simulink model "BLDC_120deg_LUT"  (R2024a)
settings: Solver=ode15s  StartTime=0.0  StopTime=1.5  RelTol=1e-3
model workspace (MAT data in the model file):
  t = 3
values from neighbouring files (symbols this model uses):
  D_m = 1e-3    (= 0.001)    [BLDC_Parameters.m]
  J_t = 1e-3    (= 0.001)    [BLDC_Parameters.m]
  L_ss = tau_s * r_s    (= 0.0003657)    [BLDC_Parameters.m]
  lambda_m = torque_const/(3*P/4)    (= 0.00985)    [BLDC_Parameters.m]
  omega = out.omega(end)    [filter.m]
  P = 8    [BLDC_Parameters.m]
  r_s = r_pp/2    (= 0.345)    [BLDC_Parameters.m]
  R_vs = 1e6    (= 1000000)    [BLDC_Parameters.m]
  tau_s = 1.06e-3    (= 0.00106)    [BLDC_Parameters.m]
  V_bus = 12    [BLDC_Parameters.m]
undefined symbols (not defined in the file or in its folder): HallError1, HallError2, HallError3, tau_corr1, WrappedHallError1
libraries: simulink x14, spsMosfetLib x6, spsSeriesRLCBranchLib x4, spsVoltageMeasurementLib x3, spsControlledCurrentSourceLib x3, slpidlib x1, spsPWMGeneratorDCDCLib x1, spsDCVoltageSourceLib x1, sps_lib x1
settings Model: Creator=matthewhasman  LastModifiedBy=matthewhasman

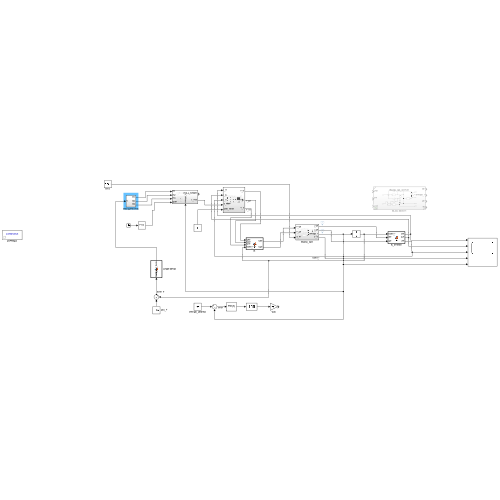
[thumbnail: Simulink's stored preview of the top-level diagram]
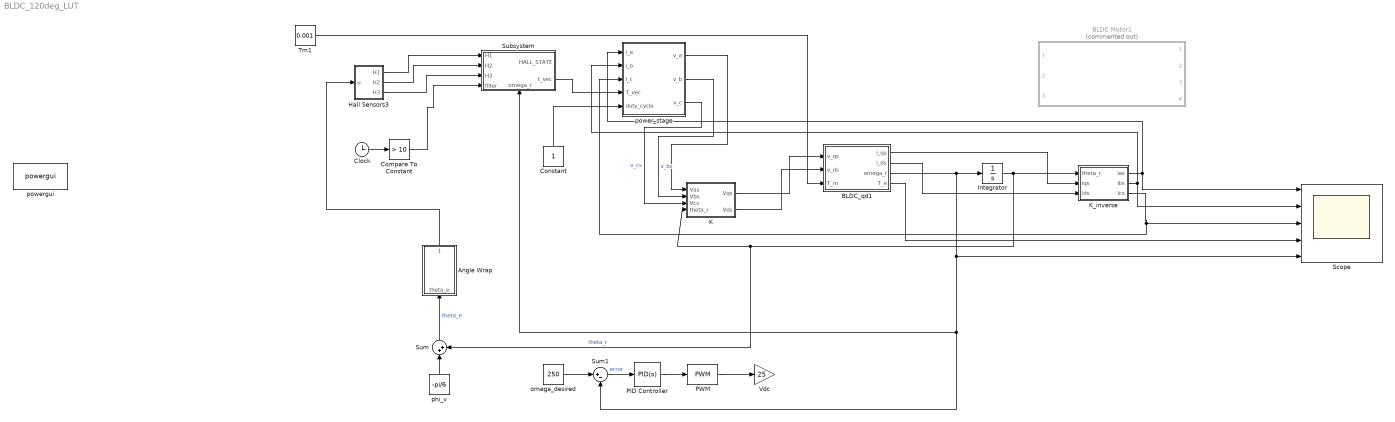
== system BLDC_120deg_LUT ==
  Angle Wrap : MATLAB Function  TreatAsAtomicUnit=on
  BLDC Motor1 : Subsystem  Commented=on  ReferencedSubsystem=BLDC_qd_coords
  BLDC_qd1 : Subsystem
  Clock : Clock
  Compare To Constant : simulink/Logic and Bit Operations/Compare To Constant  relop=>  const=10  OutDataTypeStr=boolean
  Constant : Constant
  Hall Sensors3 : Subsystem
  Integrator : Integrator
  K : MATLAB Function  TreatAsAtomicUnit=on
  K_inverse : MATLAB Function  TreatAsAtomicUnit=on
  PID Controller : slpidlib/PID Controller  Controller=PID  Form=Parallel  TimeDomain=Continuous-time  UseExternalTs=off  SampleTime=-1  IntegratorMethod=Forward Euler  FilterMethod=Forward Euler  ControllerParametersSource=internal  P=8  I=5  UseKiTs=off  D=1  UseExternalDerivativeSource=off  N=100  UseFilter=on  TunerSelectOption=Transfer Function Based (PID Tuner App)  InitialConditionSource=internal  InitialConditionForIntegrator=0  InitialConditionForFilter=0  DifferentiatorICPrevScaledInput=0  ExternalReset=none  TrackingMode=off  Kt=1  LimitOutput=off  SatLimitsSource=internal  UpperSaturationLimit=inf  LowerSaturationLimit=-inf  LinearizeAsGain=on  AntiWindupMode=none  Kb=1  LimitIntegrator=off  UpperIntegratorSaturationLimit=inf  LowerIntegratorSaturationLimit=-inf  POutMin=[]  POutMax=[]  IOutMin=[]  IOutMax=[]  DOutMin=[]  DOutMax=[]  NOutMin=[]  NOutMax=[]  SumOutMin=[]  SumOutMax=[]  SaturationOutMin=[]  SaturationOutMax=[]  PParamMin=[]  PParamMax=[]  IParamMin=[]  IParamMax=[]  DParamMin=[]  DParamMax=[]  NParamMin=[]  NParamMax=[]  KbParamMin=[]  KbParamMax=[]  KtParamMin=[]  KtParamMax=[]  KbOutMin=[]  KbOutMax=[]  KtOutMin=[]  KtOutMax=[]  IntegratorOutMin=[]  IntegratorOutMax=[]  FilterOutMin=[]  FilterOutMax=[]  SumI1OutMin=[]  SumI1OutMax=[]  SumI2OutMin=[]  SumI2OutMax=[]  SumI3OutMin=[]  SumI3OutMax=[]  SumI4OutMin=[]  SumI4OutMax=[]  SumDOutMin=[]  SumDOutMax=[]  DifferentiatorOutMin=[]  DifferentiatorOutMax=[]  FilterDiffOutCoefMin=[]  FilterDiffOutCoefMax=[]  ReciprocalOutMin=[]  ReciprocalOutMax=[]  SumDenOutMin=[]  SumDenOutMax=[]  SumNumOutMin=[]  SumNumOutMax=[]  DivideOutMin=[]  DivideOutMax=[]  UdiffTsProdOutMin=[]  UdiffTsProdOutMax=[]  NTsProdOutMin=[]  NTsProdOutMax=[]  UintegralTsProdOutMin=[]  UintegralTsProdOutMax=[]  UngainTsProdOutMin=[]  UngainTsProdOutMax=[]  ClampingZeroOutDataTypeStr=Inherit: Inherit via back propagation  ClampingZeroOutMin=[]  ClampingZeroOutMax=[]  FilterDenConstantOutDataTypeStr=Inherit: Inherit via back propagation  FilterDenConstantOutMin=[]  FilterDenConstantOutMax=[]  PCopyOutDataTypeStr=Inherit: Inherit via back propagation  PCopyOutMin=[]  PCopyOutMax=[]  NCopyOutDataTypeStr=Inherit: Inherit via back propagation  NCopyOutMin=[]  NCopyOutMax=[]  IntegratorContinuousStateAttributes=''  IntegratorStateMustResolveToSignalObject=off  IntegratorRTWStateStorageClass=Auto  FilterContinuousStateAttributes=''  FilterStateMustResolveToSignalObject=off  FilterRTWStateStorageClass=Auto  ParallelPVariant=InternalParameters  IdealPVariant=Disabled  IVariant=InternalParameters  DVariant=InternalParameters  IntegratorVariant=Continuous  SatVariant=Disabled  AWVariant=Passthrough  PCopyVariant=Disabled  TRVariant=Disabled  FdbkBlocksVariant=Forward  IdealPFdbkVariant=Disabled  SatFdbkVariant=Disabled  DerivativeFilterVariant=ContFilter  NVariant=InternalParameters  NCopyVariant=Disabled  FilterICVariant=InternalICsFilter  IntegratorICVariant=InternalICs  ExternalResetVariant=Disabled  TRSumVariant=Passthrough  SumFdbkVariant=Disabled  SumVariant=Sum_PID  TsampFilterVariant=InternalTs  TsampNgainVariant=Passthrough  TsampIntegralVariant=Disabled_SignalSpec  ExternalSaturationOutDataTypeStr=Inherit: Same as second input  DerivativeSourceVariant=ErrorSignal
  PWM : simulink/Discontinuities/PWM  DisableCoverage=on  Period=0.0001  InitialDelay=0  DisallowZeroDutyCycle=off  RunAtFixedTimeIntervals=off  SampleTime=0.1
  Scope : Scope  NumInputPorts=5
  Subsystem : Subsystem
      settings: PortSchema="{\"entries\":[{\"content\":{\"sides\":[{\"content\":{\"connectorIds\":[\"In1\",\"In2\",\"In3\",\"In4\"]},\"type\":\"ConnectorPlacement.EquallySpacedRectSide\",\"uuid\":\"971d0d47-82fe-4afe-af38-e6db618daf70\"},{\"content\":{\"connectorIds\":[\"Out1\",\"Out2\"],\"side\":\"RIGHT\"},\"type\":\"ConnectorPlacement.EquallySpacedRectSide\",\"uuid\":\"04121426-e5e1-4fdf-a823-1b0728fc829c\"},{\"content\":{\"side\":\"TOP\"},\"type\":\"ConnectorPlacement.EquallySpacedRectSide\",\"uuid\":\"8184400a-788f-412d-9776-29e4a0174c8c\"},{\"content\":{\"connectorIds\":[\"In5\"],\"side\":\"BOTTOM\"},\"type\":\"ConnectorPlacement.EquallySpacedRectSide\",\"uuid\":\"7ee8c5a1-7866-4d62-ba50-cd64eb02da7d\"}]},\"type\":\"ConnectorPlacement.EquallySpacedConnector\",\"uuid\":\"0b8e8def-6998-42e4-af89-aa5c552bf5ba\"}],\"packageUris\":[\"http://schema.mathworks.com/mf0/Connector/R2020b\"],\"version\":\"1.0\"}"
  Sum : Sum  Inputs=|++
  Sum1 : Sum  Inputs=|+-
  Tm1 : Constant  Value=0.001
  Vdc : Gain  Gain=25
  omega_desired : Constant  Value=250
  phi_v : Constant  Value=-pi/6
  power_stage : Subsystem
  powergui : sps_lib/powergui  Priority=1  SimulationMode=Continuous  SampleTime=50e-6  frequency=60  Iterations=50  frequencyindice=0  Pbase=100e6  ErrMax=1e-4  UnitsV=kV  UnitsW=MW  buscounter=0  FunctionMessages=off  echomessages=off  EnableUseOfTLC=off  CurrentSourceSwitches=off  DisableSnubberDevices=off  DisableRonSwitches=off  DisableVfSwitches=off  DisplayEquations=off  AutomaticDiscreteSolvers=off  SolverType=Tustin/Backward Euler (TBE)  Interpol=off  ExternalGateDelay=off  methode=off  Ts=100  x0status=blocks  SPID=on  SwTol=0  HookPort=off  NonlinearTolerance=1e-4  nMaxIteration=100  ContinueOnMaxIteration=off  RestoreLinks=warning  ResistiveCurrentMeasurement=off  Frange=[0:2:500]  Ylog=off  Xlog=on  ShowGrid=off  save=off  variable=ZData  structure=0  ZoomFFT=off  StartTime=0.0  cycles=1  DisplayStyle=1  fundamental=60  FreqAxis=off  MaxFrequency=1000  frequencyindicesteady=1  RmsSteady=1  display=off
  wires:
  Integrator/1 -> K_inverse/1(theta_r), K/4(theta_r), Sum/2  "theta_r"
  BLDC_qd1/1(i_qs) -> K_inverse/2(iqs)
  BLDC_qd1/2(i_ds) -> K_inverse/3(ids)
  K/1(Vqs) -> BLDC_qd1/1(v_qs)
  Tm1/1 -> BLDC_qd1/3(T_m)
  phi_v/1 -> Sum/1
  omega_desired/1 -> Sum1/1
  Sum1/1 -> PID Controller/1  "error"
  PID Controller/1 -> PWM/1
  PWM/1 -> Vdc/1
  K/2(Vds) -> BLDC_qd1/2(v_ds)
  Sum/1 -> Angle Wrap/1(theta_e)  "theta_e"
  BLDC_qd1/3(omega_r) -> Subsystem/5(omega_r), Sum1/2, Scope/5, Integrator/1
  BLDC_qd1/4(T_e) -> Scope/4
  K_inverse/1(ias) -> power_stage/1(i_a), Scope/1
  K_inverse/2(ibs) -> power_stage/2(i_b), Scope/2
  K_inverse/3(ics) -> power_stage/3(i_c), Scope/3
  Constant/1 -> power_stage/5(duty_cycle)
  power_stage/1(v_a) -> K/1(Vas)
  power_stage/2(v_b) -> K/2(Vbs)  "v_bs"
  power_stage/3(v_c) -> K/3(Vcs)  "v_cs"
  Angle Wrap/1(wrapped_theta) -> Hall Sensors3/1(u)
  Clock/1 -> Compare To Constant/1
  Hall Sensors3/1(H1) -> Subsystem/1(H1)
  Hall Sensors3/2(H2) -> Subsystem/2(H2)
  Hall Sensors3/3(H3) -> Subsystem/3(H3)
  Compare To Constant/1 -> Subsystem/4(filter)
  Subsystem/2(t_vec) -> power_stage/4(T_vec)

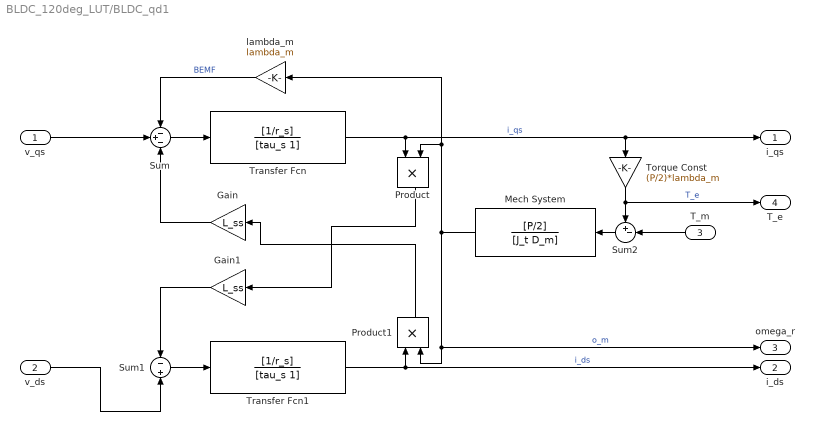
== system BLDC_120deg_LUT/BLDC_qd1 ==
  v_qs : Inport
  v_ds : Inport  Port=2
  T_m : Inport  Port=3
  Gain : Gain  Gain=L_ss
  Gain1 : Gain  Gain=L_ss
  Mech System : TransferFcn  Numerator=[P/2]  Denominator=[J_t D_m]
  Product : Product
  Product1 : Product
  Sum : Sum  Inputs=-+-
  Sum1 : Sum  Inputs=-+
  Sum2 : Sum  Inputs=+-|
  Torque Const : Gain  Gain=(P/2)*lambda_m
  Transfer Fcn : TransferFcn  Numerator=[1/r_s]  Denominator=[tau_s 1]
  Transfer Fcn1 : TransferFcn  Numerator=[1/r_s]  Denominator=[tau_s 1]
  lambda_m : Gain  Gain=lambda_m
  i_qs : Outport
  i_ds : Outport  Port=2
  omega_r : Outport  Port=3
  T_e : Outport  Port=4
  wires:
  T_m/1 -> Sum2/2
  Sum1/1 -> Transfer Fcn1/1
  Gain1/1 -> Sum1/1
  Product1/1 -> Gain/1
  Transfer Fcn1/1 -> i_ds/1, Product1/1  "i_ds"
  Mech System/1 -> lambda_m/1, Product/2, omega_r/1, Product1/2  "o_m"
  Torque Const/1 -> T_e/1, Sum2/1  "T_e"
  v_ds/1 -> Sum1/2
  Transfer Fcn/1 -> i_qs/1, Torque Const/1, Product/1  "i_qs"
  Product/1 -> Gain1/1
  Gain/1 -> Sum/3
  v_qs/1 -> Sum/2
  Sum/1 -> Transfer Fcn/1
  Sum2/1 -> Mech System/1
  lambda_m/1 -> Sum/1  "BEMF"

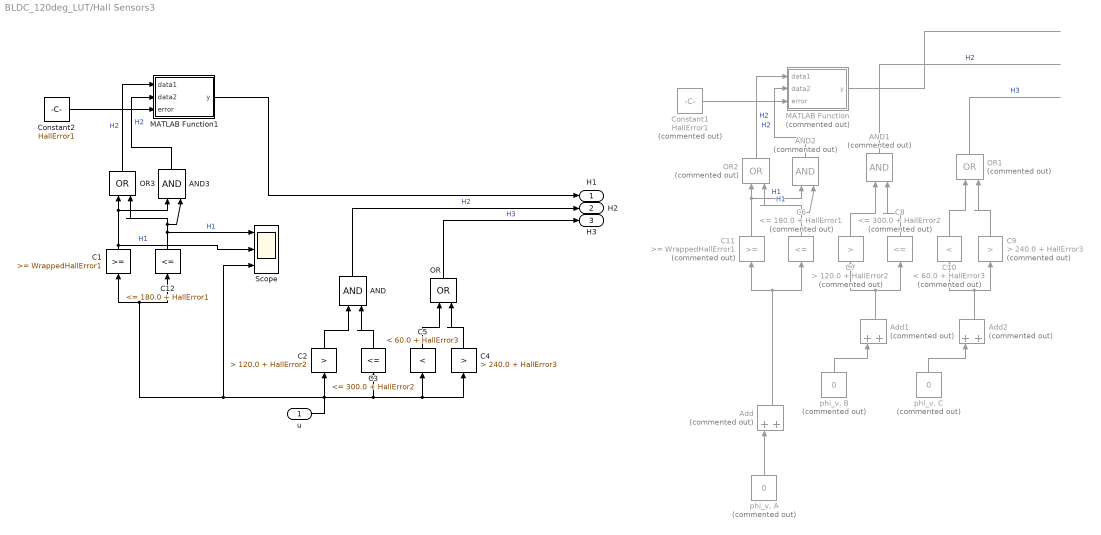
== system BLDC_120deg_LUT/Hall Sensors3 ==
  u : Inport
  AND : Logic  IconShape=distinctive  AllPortsSameDT=off  OutDataTypeStr=boolean
  AND1 : Logic  Commented=on  IconShape=distinctive  AllPortsSameDT=off  OutDataTypeStr=boolean
  AND2 : Logic  Commented=on  IconShape=distinctive  AllPortsSameDT=off  OutDataTypeStr=boolean
  AND3 : Logic  IconShape=distinctive  AllPortsSameDT=off  OutDataTypeStr=boolean
  Add : Sum  Commented=on
  Add1 : Sum  Commented=on
  Add2 : Sum  Commented=on
  C1 : simulink/Logic and Bit Operations/Compare To Constant  relop=>=  const=WrappedHallError1  OutDataTypeStr=boolean
  C10 : simulink/Logic and Bit Operations/Compare To Constant  Commented=on  relop=<  const=60.0 + HallError3  OutDataTypeStr=boolean
  C11 : simulink/Logic and Bit Operations/Compare To Constant  Commented=on  relop=>=  const=WrappedHallError1  OutDataTypeStr=boolean
  C12 : simulink/Logic and Bit Operations/Compare To Constant  relop=<=  const=180.0 + HallError1  OutDataTypeStr=boolean
  C2 : simulink/Logic and Bit Operations/Compare To Constant  relop=>  const=120.0 + HallError2  OutDataTypeStr=boolean
  C3 : simulink/Logic and Bit Operations/Compare To Constant  relop=<=  const=300.0 + HallError2  OutDataTypeStr=boolean
  C4 : simulink/Logic and Bit Operations/Compare To Constant  relop=>  const=240.0 + HallError3  OutDataTypeStr=boolean
  C5 : simulink/Logic and Bit Operations/Compare To Constant  relop=<  const=60.0 + HallError3  OutDataTypeStr=boolean
  C6 : simulink/Logic and Bit Operations/Compare To Constant  Commented=on  relop=<=  const=180.0 + HallError1  OutDataTypeStr=boolean
  C7 : simulink/Logic and Bit Operations/Compare To Constant  Commented=on  relop=>  const=120.0 + HallError2  OutDataTypeStr=boolean
  C8 : simulink/Logic and Bit Operations/Compare To Constant  Commented=on  relop=<=  const=300.0 + HallError2  OutDataTypeStr=boolean
  C9 : simulink/Logic and Bit Operations/Compare To Constant  Commented=on  relop=>  const=240.0 + HallError3  OutDataTypeStr=boolean
  Constant1 : Constant  Commented=on  Value=HallError1
  Constant2 : Constant  Value=HallError1
  MATLAB Function : MATLAB Function  Commented=on  TreatAsAtomicUnit=on
  MATLAB Function1 : MATLAB Function  TreatAsAtomicUnit=on
  OR : Logic  Operator=OR  IconShape=distinctive  AllPortsSameDT=off  OutDataTypeStr=boolean
  OR1 : Logic  Commented=on  Operator=OR  IconShape=distinctive  AllPortsSameDT=off  OutDataTypeStr=boolean
  OR2 : Logic  Commented=on  Operator=OR  IconShape=distinctive  AllPortsSameDT=off  OutDataTypeStr=boolean
  OR3 : Logic  Operator=OR  IconShape=distinctive  AllPortsSameDT=off  OutDataTypeStr=boolean
  Scope : Scope  NumInputPorts=3
  "phi_v, A" : Constant  Commented=on  Value=0
  "phi_v, B" : Constant  Commented=on  Value=0
  "phi_v, C" : Constant  Commented=on  Value=0
  H1 : Outport
  H2 : Outport  Port=2
  H3 : Outport  Port=3
  wires:
  C5/1 -> OR/1
  AND/1 -> H2/1  "H2"
  C4/1 -> OR/2
  C3/1 -> AND/2
  C2/1 -> AND/1
  OR/1 -> H3/1  "H3"
  Add1/1 -> C8/1, C7/1
  "phi_v, C"/1 -> Add2/1
  "phi_v, B"/1 -> Add1/1
  C10/1 -> OR1/1
  ? -> Add2/2, Add1/2, Add/2
  OR2/1 -> MATLAB Function/1(data1)  "H2"
  "phi_v, A"/1 -> Add/1
  C9/1 -> OR1/2
  Add/1 -> C6/1, C11/1
  C7/1 -> AND1/1
  Add2/1 -> C10/1, C9/1
  Constant1/1 -> MATLAB Function/3(error)
  OR1/1 -> ?  "H3"
  AND1/1 -> ?  "H2"
  C6/1 -> AND2/2, OR2/2  "H1"
  AND2/1 -> MATLAB Function/2(data2)  "H2"
  MATLAB Function/1(y) -> ?
  C11/1 -> AND2/1, OR2/1  "H1"
  C8/1 -> AND1/2
  u/1 -> Scope/3, C12/1, C1/1, C2/1, C5/1, C4/1, C3/1
  OR3/1 -> MATLAB Function1/1(data1)  "H2"
  Constant2/1 -> MATLAB Function1/3(error)
  C1/1 -> AND3/1, OR3/1, Scope/2  "H1"
  C12/1 -> AND3/2, OR3/2, Scope/1  "H1"
  AND3/1 -> MATLAB Function1/2(data2)  "H2"
  MATLAB Function1/1(y) -> H1/1

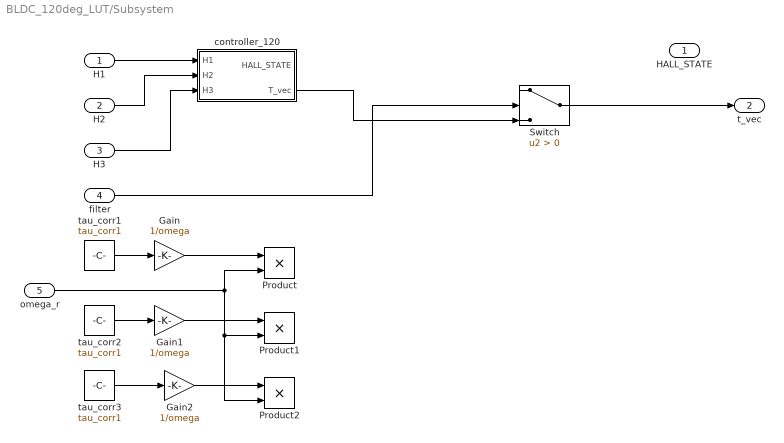
== system BLDC_120deg_LUT/Subsystem ==
  H1 : Inport
  H2 : Inport  Port=2
  H3 : Inport  Port=3
  filter : Inport  Port=4
  omega_r : Inport  Port=5
  Gain : Gain  Gain=1/omega
  Gain1 : Gain  Gain=1/omega
  Gain2 : Gain  Gain=1/omega
  Product : Product
  Product1 : Product
  Product2 : Product
  Switch : Switch  Criteria=u2 > Threshold  SaturateOnIntegerOverflow=off  InputSameDT=off
  controller_120 : MATLAB Function  TreatAsAtomicUnit=on
  tau_corr1 : Constant  Value=tau_corr1
  tau_corr2 : Constant  Value=tau_corr1
  tau_corr3 : Constant  Value=tau_corr1
  HALL_STATE : Outport
  t_vec : Outport  Port=2
  wires:
  H1/1 -> controller_120/1(H1)
  H2/1 -> controller_120/2(H2)
  H3/1 -> controller_120/3(H3)
  filter/1 -> Switch/2
  Switch/1 -> t_vec/1
  controller_120/2(T_vec) -> Switch/3
  tau_corr1/1 -> Gain/1
  Gain/1 -> Product/1
  tau_corr2/1 -> Gain1/1
  tau_corr3/1 -> Gain2/1
  Gain1/1 -> Product1/1
  Gain2/1 -> Product2/1
  omega_r/1 -> Product2/2, Product1/2, Product/2

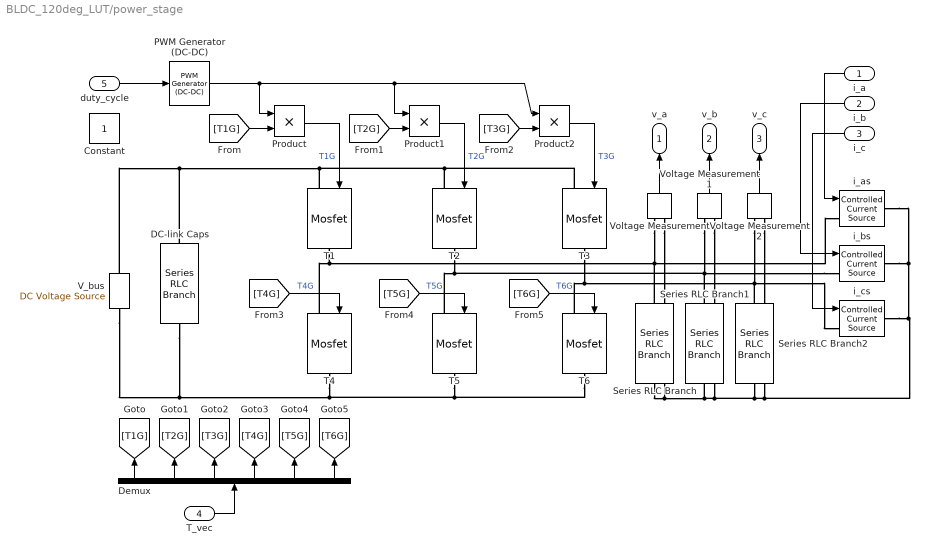
== system BLDC_120deg_LUT/power_stage ==
  i_a : Inport
  i_b : Inport  Port=2
  i_c : Inport  Port=3
  T_vec : Inport  Port=4
  duty_cycle : Inport  Port=5
  Constant : Constant
  DC-link Caps : spsSeriesRLCBranchLib/Series RLC Branch  LConnTagsString=__new0  RConnTagsString=__new0  BranchType=RC  Resistance=1e-6  Inductance=0  SetiL0=off  InitialCurrent=0  Capacitance=100e-6  Setx0=off  InitialVoltage=0  Measurements=None
  Demux : Demux  Outputs=6
  PWM Generator (DC-DC) : spsPWMGeneratorDCDCLib/PWM Generator (DC-DC)  Fsw=f_SW_Hz  Ts=0
  Product : Product
  Product1 : Product
  Product2 : Product
  Series RLC Branch : spsSeriesRLCBranchLib/Series RLC Branch  LConnTagsString=__new0  RConnTagsString=__new0  BranchType=R  Resistance=R_vs  Inductance=0  SetiL0=off  InitialCurrent=0  Capacitance=inf  Setx0=off  InitialVoltage=0  Measurements=None
  Series RLC Branch1 : spsSeriesRLCBranchLib/Series RLC Branch  LConnTagsString=__new0  RConnTagsString=__new0  BranchType=R  Resistance=R_vs  Inductance=0  SetiL0=off  InitialCurrent=0  Capacitance=inf  Setx0=off  InitialVoltage=0  Measurements=None
  Series RLC Branch2 : spsSeriesRLCBranchLib/Series RLC Branch  LConnTagsString=__new0  RConnTagsString=__new0  BranchType=R  Resistance=R_vs  Inductance=0  SetiL0=off  InitialCurrent=0  Capacitance=inf  Setx0=off  InitialVoltage=0  Measurements=None
  T{1..6} (6 alike) : spsMosfetLib/Mosfet  Ron=R_dsON_Ohm  Lon=0  Rd=0.01  Vfd=0.7  IC=0  Rs=1e5  Cs=inf  Measurements=off
  V_bus : spsDCVoltageSourceLib/DC Voltage Source  Amplitude=V_bus  Measurements=None
  Voltage Measurement : spsVoltageMeasurementLib/Voltage Measurement  PhasorSimulation=off  OutputType=Complex  PSBequivalent=0
  Voltage Measurement1 : spsVoltageMeasurementLib/Voltage Measurement  PhasorSimulation=off  OutputType=Complex  PSBequivalent=0
  Voltage Measurement2 : spsVoltageMeasurementLib/Voltage Measurement  PhasorSimulation=off  OutputType=Complex  PSBequivalent=0
  i_as : spsControlledCurrentSourceLib/Controlled Current Source  Initialize=on  Source_Type=AC  Amplitude=0  Phase=0  Frequency=0  Measurements=None
  i_bs : spsControlledCurrentSourceLib/Controlled Current Source  Initialize=on  Source_Type=AC  Amplitude=0  Phase=0  Frequency=0  Measurements=None
  i_cs : spsControlledCurrentSourceLib/Controlled Current Source  Initialize=on  Source_Type=AC  Amplitude=0  Phase=0  Frequency=0  Measurements=None
  v_a : Outport
  v_b : Outport  Port=2
  v_c : Outport  Port=3
  wires:
  T_vec/1 -> Demux/1
  Product1/1 -> T2/1  "T2G"
  PWM Generator (DC-DC)/1 -> Product/1, Product2/1, Product1/1
  Demux/6 -> [T6G]
  [T4G] -> T4/1  "T4G"
  [T5G] -> T5/1  "T5G"
  Demux/4 -> [T4G]
  Voltage Measurement/1 -> v_a/1
  [T2G] -> Product1/2
  Voltage Measurement1/1 -> v_b/1
  Voltage Measurement2/1 -> v_c/1
  i_a/1 -> i_as/1
  Demux/1 -> [T1G]
  Demux/5 -> [T5G]
  [T6G] -> T6/1  "T6G"
  i_c/1 -> i_cs/1
  Product/1 -> T1/1  "T1G"
  [T3G] -> Product2/2
  i_b/1 -> i_bs/1
  Product2/1 -> T3/1  "T3G"
  Demux/2 -> [T2G]
  Demux/3 -> [T3G]
  [T1G] -> Product/2
  duty_cycle/1 -> PWM Generator (DC-DC)/1
  connections:
  i_bs/LConn1 -- Voltage Measurement1/LConn1 -- Series RLC Branch1/LConn1 -- T2/RConn1 -- T5/LConn1
  DC-link Caps/RConn1 -- V_bus/LConn1 -- T4/RConn1 -- T6/RConn1 -- T5/RConn1
  DC-link Caps/LConn1 -- V_bus/RConn1 -- T1/LConn1 -- T3/LConn1 -- T2/LConn1
  T4/LConn1 -- T1/RConn1 -- Voltage Measurement/LConn1 -- Series RLC Branch/LConn1 -- i_as/LConn1
  T3/RConn1 -- T6/LConn1 -- Voltage Measurement2/LConn1 -- Series RLC Branch2/LConn1 -- i_cs/LConn1
  Series RLC Branch/RConn1 -- Voltage Measurement/LConn2 -- i_bs/RConn1 -- i_as/RConn1 -- i_cs/RConn1 -- Voltage Measurement2/LConn2 -- Series RLC Branch2/RConn1 -- Voltage Measurement1/LConn2 -- Series RLC Branch1/RConn1

== matlab function BLDC_120deg_LUT/K ==
  data: Vas input; Vqs output; Vbs input; Vcs input; Vds output; theta_r input
function [Vqs, Vds] = fcn(Vas, Vbs, Vcs, theta_r)
offset = 2*pi/3;
k = (2/3)*[cos(theta_r), cos(theta_r - offset), cos(theta_r + offset);
           sin(theta_r), sin(theta_r - offset), sin(theta_r + offset)];

qds_voltage = k * [Vas; Vbs; Vcs];

Vqs = qds_voltage(1);
Vds = qds_voltage(2);

end

== matlab function BLDC_120deg_LUT/K_inverse ==
  data: theta_r input; ias output; iqs input; ids input; ibs output; ics output
function [ias, ibs, ics] = fcn(theta_r, iqs, ids)
offset = 2*pi/3;
k_inverse = [cos(theta_r), sin(theta_r);
             cos(theta_r - offset), sin(theta_r - offset);
             cos(theta_r + offset), sin(theta_r + offset)];

abc_currents = k_inverse * [iqs; ids];

ias = abc_currents(1);
ibs = abc_currents(2);
ics = abc_currents(3);

end

== matlab function BLDC_120deg_LUT/Angle Wrap ==
  data: theta_e input; wrapped_theta output
function wrapped_theta = fcn(theta_e)

wrapped_theta = wrapTo2Pi(theta_e) * 180 / pi;

== matlab function BLDC_120deg_LUT/Hall Sensors3/MATLAB Function1 ==
  data: data1 input; y output; data2 input; error input
function y = fcn(data1, data2, error)

if error > 0
    y = data2;

else 
    y = data1;

end

== matlab function BLDC_120deg_LUT/Subsystem/controller_120 ==
  data: H1 input; HALL_STATE output; H2 input; H3 input; T_vec output
function [HALL_STATE, T_vec] = controller_6step_120_sim(H1,H2,H3)
[HALL_STATE, T_vec] = controller_6step_120(H1,H2,H3);
end

== matlab function BLDC_120deg_LUT/Hall Sensors3/MATLAB Function ==
  data: data1 input; y output; data2 input; error input
function y = fcn(data1, data2, error)

if error > 0
    y = data2;

else 
    y = data1;

end
